simulink subsystem "A"  (R2024a)
settings: Solver=VariableStepAuto  StartTime=0.0  StopTime=1000.0  RelTol=1e-3
undefined symbols (not defined in the file): A_deltaAxio
settings Model: DefaultTestHarness=A_Harness  Creator=nicol  LastModifiedBy=nicol

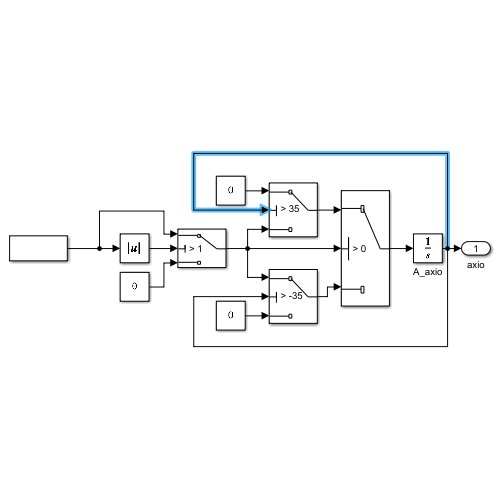
[thumbnail: Simulink's stored preview of the top-level diagram]
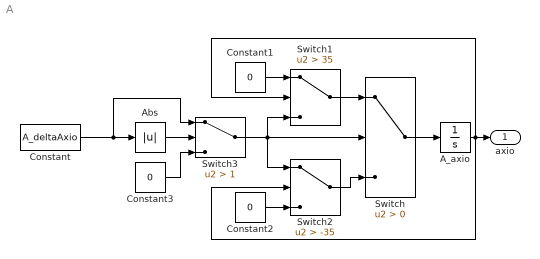
== system A ==
  A_axio : Integrator
  Abs : Abs  SaturateOnIntegerOverflow=off
  Constant : Constant  Value=A_deltaAxio
  Constant1 : Constant  Value=0
  Constant2 : Constant  Value=0
  Constant3 : Constant  Value=0
  Switch : Switch  Criteria=u2 > Threshold  SaturateOnIntegerOverflow=off  InputSameDT=off
  Switch1 : Switch  Criteria=u2 > Threshold  Threshold=35  SaturateOnIntegerOverflow=off  InputSameDT=off
  Switch2 : Switch  Criteria=u2 > Threshold  Threshold=-35  SaturateOnIntegerOverflow=off  InputSameDT=off
  Switch3 : Switch  Criteria=u2 > Threshold  Threshold=1  SaturateOnIntegerOverflow=off  InputSameDT=off
  axio : Outport
  wires:
  Constant1/1 -> Switch1/1
  Constant2/1 -> Switch2/3
  A_axio/1 -> Switch1/2, Switch2/2, axio/1
  Switch1/1 -> Switch/1
  Switch/1 -> A_axio/1
  Constant/1 -> Abs/1, Switch3/1
  Switch2/1 -> Switch/3
  Switch3/1 -> Switch/2, Switch1/3, Switch2/1
  Abs/1 -> Switch3/2
  Constant3/1 -> Switch3/3
